simulink model "Soft_actuator_master_2021"  (R2020b)
settings: Solver=FixedStepAuto  StartTime=0.0  StopTime=inf  FixedStep=Ts  RelTol=1e-3  EnableMultiTasking=on
undefined symbols (not defined in the file or in its folder): Ts
libraries: arduinolib x6, simulink x2, pid_lib x1, dspfdesign x1
settings Model: SimulationMode=external  SILPILModeSetting=veronly  ExtModeTrigDuration=2  Creator=4D Lab  LastModifiedBy=Jakob Jansson
settings SolverCC: PositivePriorityOrder=on
settings OptimizationCC: EnhancedBackFolding=on  PassReuseOutputArgsAs=Individual arguments  ZeroExternalMemoryAtStartup=off  ZeroInternalMemoryAtStartup=off  MaxStackSize=64  OptimizeBlockOrder=speed  DifferentSizesBufferReuse=on  OptimizationCustomize=off  EfficientTunableParamExpr=on
settings DebuggingCC: ParameterTunabilityLossMsg=error
settings HardwareCC: ProdBitPerInt=16  ProdBitPerPointer=16  ProdBitPerSizeT=16  ProdBitPerPtrDiffT=16  ProdLargestAtomicFloat=None  ProdWordSize=8  ProdHWDeviceType=Atmel->AVR
settings RTWCC: Description=Embedded Coder  SystemTargetFile=ert.tlc  HardwareBoard=Arduino Mega 2560  TLCOptions="-aInlineSetEventsForThisBaseRateFcn=TLC_FALSE -aSuppressMultiTaskScheduler=TLC_FALSE   -aRateBasedStepFcn=1"  TemplateMakefile=ert_default_tmf  Toolchain=Arduino AVR  BuildConfiguration=Faster Runs
settings CodeAppCC: ForceParamTrailComments=on  IgnoreCustomStorageClasses=off  OperatorAnnotations=on  SimulinkDataObjDesc=on  SFDataObjDesc=on  InsertBlockDesc=on
settings ERTTargetCC: SupportContinuousTime=on  SupportVariableSizeSignals=on  ExtMode=on  ExtModeStaticAllocSize=2048  ExtModeMexArgs='127.0.0.1' 0 17725

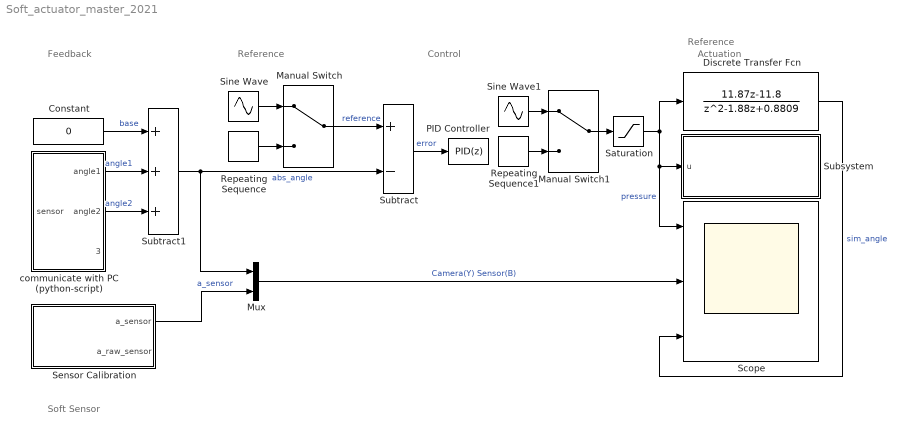
== system Soft_actuator_master_2021 ==
  note: Reference
  note: Feedback
  note: Soft Sensor
  note: Reference
  note: Actuation
  note: Control
  Constant : Constant  Value=0
  Discrete Transfer Fcn : DiscreteTransferFcn  Numerator=[11.87 -11.8]  Denominator=[1 -1.88 0.8809]
  Manual Switch : ManualSwitch
  Manual Switch1 : ManualSwitch
  Mux : Mux  Inputs=2
  PID Controller : pid_lib/PID Controller  Controller=PID  Form=Parallel  TimeDomain=Discrete-time  UseExternalTs=off  SampleTime=-1  IntegratorMethod=Forward Euler  FilterMethod=Forward Euler  ControllerParametersSource=internal  P=0.014114  I=0.11  D=-7.28e-05  UseFilter=on  N=25.7343  TunerSelectOption=Transfer Function Based (PID Tuner App)  InitialConditionSource=internal  InitialConditionForIntegrator=0  InitialConditionForFilter=0  DifferentiatorICPrevScaledInput=0  ExternalReset=none  TrackingMode=off  Kt=1  LimitOutput=off  SatLimitsSource=internal  UpperSaturationLimit=inf  LowerSaturationLimit=-inf  LinearizeAsGain=on  AntiWindupMode=none  Kb=1  POutMin=[]  POutMax=[]  IOutMin=[]  IOutMax=[]  DOutMin=[]  DOutMax=[]  NOutMin=[]  NOutMax=[]  SumOutMin=[]  SumOutMax=[]  SaturationOutMin=[]  SaturationOutMax=[]  PParamMin=[]  PParamMax=[]  IParamMin=[]  IParamMax=[]  DParamMin=[]  DParamMax=[]  NParamMin=[]  NParamMax=[]  KbParamMin=[]  KbParamMax=[]  KtParamMin=[]  KtParamMax=[]  KbOutMin=[]  KbOutMax=[]  KtOutMin=[]  KtOutMax=[]  IntegratorOutMin=[]  IntegratorOutMax=[]  FilterOutMin=[]  FilterOutMax=[]  SumI1OutMin=[]  SumI1OutMax=[]  SumI2OutMin=[]  SumI2OutMax=[]  SumI3OutMin=[]  SumI3OutMax=[]  SumI4OutMin=[]  SumI4OutMax=[]  SumDOutMin=[]  SumDOutMax=[]  DifferentiatorOutMin=[]  DifferentiatorOutMax=[]  FilterDiffOutCoefMin=[]  FilterDiffOutCoefMax=[]  ReciprocalOutMin=[]  ReciprocalOutMax=[]  SumDenOutMin=[]  SumDenOutMax=[]  SumNumOutMin=[]  SumNumOutMax=[]  DivideOutMin=[]  DivideOutMax=[]  UdiffTsProdOutMin=[]  UdiffTsProdOutMax=[]  NTsProdOutMin=[]  NTsProdOutMax=[]  UintegralTsProdOutMin=[]  UintegralTsProdOutMax=[]  UngainTsProdOutMin=[]  UngainTsProdOutMax=[]  IntegratorContinuousStateAttributes=''  IntegratorStateMustResolveToSignalObject=off  IntegratorRTWStateStorageClass=Auto  FilterContinuousStateAttributes=''  FilterStateMustResolveToSignalObject=off  FilterRTWStateStorageClass=Auto  ParallelPVariant=InternalParameters  IdealPVariant=Disabled  IVariant=InternalParameters  DVariant=InternalParameters  IntegratorVariant=Discrete  SatVariant=Disabled  AWVariant=Passthrough  PCopyVariant=Disabled  TRVariant=Disabled  FdbkBlocksVariant=Forward  IdealPFdbkVariant=Disabled  SatFdbkVariant=Disabled  DerivativeFilterVariant=ForwardEulerFilter  NVariant=InternalParameters  NCopyVariant=Disabled  FilterICVariant=InternalICsFilter  IntegratorICVariant=InternalICs  ExternalResetVariant=Disabled  TRSumVariant=Passthrough  SumFdbkVariant=Disabled  SumVariant=Sum_PID  TsampFilterVariant=InternalTs  TsampNgainVariant=Passthrough  TsampIntegralVariant=Passthrough  ExternalSaturationOutDataTypeStr=Inherit: Same as second input
  Repeating Sequence : simulink/Sources/Repeating Sequence  rep_seq_t=[0 4 6 10 12]  rep_seq_y=[0 0 180 180 0]
  Repeating Sequence1 : simulink/Sources/Repeating Sequence  rep_seq_t=[0 4 6 10 12]  rep_seq_y=[0 0 180 180 0]
  Saturation : Saturate  UpperLimit=6  LowerLimit=0
  Scope : Scope  NumInputPorts=3
  Sensor Calibration : Subsystem
  Sine Wave : Sin  Amplitude=45  Bias=135  SampleTime=Ts
  Sine Wave1 : Sin  Bias=1  Frequency=2  SampleTime=Ts
  Subsystem : Subsystem
  Subtract : Sum  Inputs=+-
  Subtract1 : Sum  Inputs=+++
  communicate with PC (python-script) : Subsystem
  wires:
  Subtract1/1 -> Subtract/2, Mux/1  "abs_angle"
  Subtract/1 -> PID Controller/1  "error"
  Sine Wave/1 -> Manual Switch/1
  Repeating Sequence/1 -> Manual Switch/2
  Manual Switch/1 -> Subtract/1  "reference"
  communicate with PC (python-script)/2(angle2) -> Subtract1/3  "angle2"
  communicate with PC (python-script)/1(angle1) -> Subtract1/2  "angle1"
  Constant/1 -> Subtract1/1  "base"
  Discrete Transfer Fcn/1 -> Scope/3  "sim_angle"
  Manual Switch1/1 -> Saturation/1
  Saturation/1 -> Discrete Transfer Fcn/1, Scope/1, Subsystem/1(u)  "pressure"
  Sensor Calibration/1(a_sensor) -> Mux/2  "a_sensor"
  Mux/1 -> Scope/2  "Camera(Y) Sensor(B)"
  Repeating Sequence1/1 -> Manual Switch1/2
  Sine Wave1/1 -> Manual Switch1/1

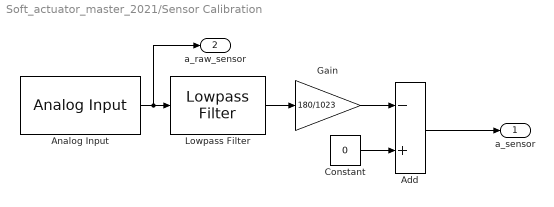
== system Soft_actuator_master_2021/Sensor Calibration ==
  Add : Sum  Inputs=-+
  Analog Input : arduinolib/Analog Input  pinNumber=4  ReadResultsOnly=off  ConversionTriggerSource=Software  ExternalTriggerType=uint32( 0 )  OutputDataType=uint16  EnableConversionCompleteNotify=off  EnableOuputStatus=off  SampleTime=Ts  blockPlatform=arduino
  Constant : Constant  Value=0
  Gain : Gain  Gain=180/1023
  Lowpass Filter : dspfdesign/Lowpass Filter  FilterType=FIR  DesignForMinimumOrder=on  FilterOrder=50  PassbandFrequency=8e3  StopbandFrequency=12e3  PassbandRipple=0.1  StopbandAttenuation=80  InheritSampleRate=off  SampleRate=44100  SimulateUsing=Interpreted execution  roundingMode=Floor  coeffsDataTypeStr=fixdt(1,16)
  a_sensor : Outport
  a_raw_sensor : Outport  Port=2
  wires:
  Gain/1 -> Add/1
  Constant/1 -> Add/2
  Analog Input/1 -> a_raw_sensor/1, Lowpass Filter/1
  Lowpass Filter/1 -> Gain/1
  Add/1 -> a_sensor/1

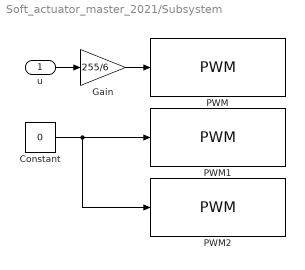
== system Soft_actuator_master_2021/Subsystem ==
  u : Inport
  Constant : Constant  Value=0
  Gain : Gain  Gain=255/6
  PWM : arduinolib/PWM  pinNumber=3  frequencyType=Default  desiredFrequency=490.2  achievableFrequency=490.2
  PWM1 : arduinolib/PWM  pinNumber=5  frequencyType=Default  desiredFrequency=490.2  achievableFrequency=490.2
  PWM2 : arduinolib/PWM  pinNumber=6  frequencyType=Default  desiredFrequency=490.2  achievableFrequency=490.2
  wires:
  Gain/1 -> PWM/1
  u/1 -> Gain/1
  Constant/1 -> PWM1/1, PWM2/1

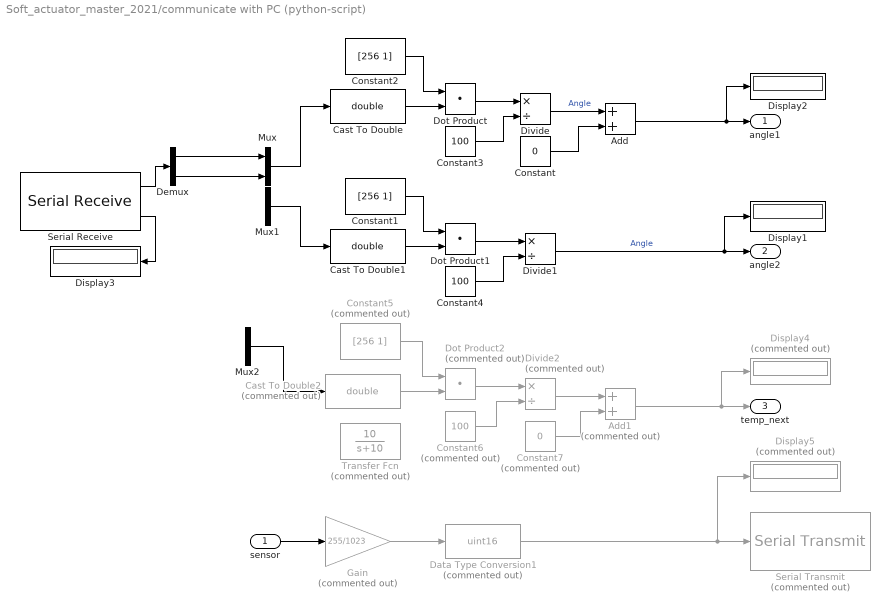
== system Soft_actuator_master_2021/communicate with PC (python-script) ==
  sensor : Inport
  Add : Sum
  Add1 : Sum  Commented=on
  Cast To Double : DataTypeConversion  OutDataTypeStr=double
  Cast To Double1 : DataTypeConversion  OutDataTypeStr=double
  Cast To Double2 : DataTypeConversion  Commented=on  OutDataTypeStr=double
  Constant : Constant  Value=0
  Constant1 : Constant  Value=[256 1]
  Constant2 : Constant  Value=[256 1]
  Constant3 : Constant  Value=100
  Constant4 : Constant  Value=100
  Constant5 : Constant  Commented=on  Value=[256 1]  OutDataTypeStr=double
  Constant6 : Constant  Commented=on  Value=100
  Constant7 : Constant  Commented=on  Value=0
  Data Type Conversion1 : DataTypeConversion  Commented=on  OutDataTypeStr=uint16
  Demux : Demux  Outputs=2
  Display1 : Display
  Display2 : Display
  Display3 : Display
  Display4 : Display  Commented=on
  Display5 : Display  Commented=on
  Divide : Product  Inputs=*/
  Divide1 : Product  Inputs=*/
  Divide2 : Product  Commented=on  Inputs=*/  OutDataTypeStr=double
  Dot Product : DotProduct  InputSameDT=on  OutDataTypeStr=Inherit: Inherit via internal rule
  Dot Product1 : DotProduct  InputSameDT=on  OutDataTypeStr=Inherit: Inherit via internal rule
  Dot Product2 : DotProduct  Commented=on  OutDataTypeStr=double  InputSameDT=on
  Gain : Gain  Commented=on  Gain=255/1023  ParamDataTypeStr=uint16
  Mux : Mux  Inputs=2
  Mux1 : Mux  Inputs=2
  Mux2 : Mux  Inputs=2
  Serial Receive : arduinolib/Serial Receive  isARMArch=off  portNumber=1  DataType=uint8  Datalength=2  SampleTime=Ts  showOutStatus=on  blockPlatform=arduino
      settings: SourceProductBaseCode=ARDUINO
  Serial Transmit : arduinolib/Serial Transmit  Commented=on  portNumber=1  sendmode=println  sendformat=Decimal  floatprecision=2  blockPlatform=arduino
  Transfer Fcn : TransferFcn  Commented=on  Numerator=[10]  Denominator=[1 10]
  angle1 : Outport  VectorParamsAs1DForOutWhenUnconnected=off
  angle2 : Outport  Port=2  VectorParamsAs1DForOutWhenUnconnected=off
  temp_next : Outport  Port=3  VectorParamsAs1DForOutWhenUnconnected=off
  wires:
  Constant3/1 -> Divide/2
  Cast To Double/1 -> Dot Product/2
  Constant2/1 -> Dot Product/1
  Dot Product/1 -> Divide/1
  Serial Receive/1 -> Demux/1
  Demux/1 -> Mux/1
  Demux/2 -> Mux/2
  Dot Product1/1 -> Divide1/1
  Constant4/1 -> Divide1/2
  Cast To Double1/1 -> Dot Product1/2
  Constant1/1 -> Dot Product1/1
  Mux/1 -> Cast To Double/1
  Mux1/1 -> Cast To Double1/1
  Divide1/1 -> Display1/1, angle2/1  "Angle"
  Serial Receive/2 -> Display3/1
  Cast To Double2/1 -> Dot Product2/2
  Constant5/1 -> Dot Product2/1
  Constant6/1 -> Divide2/2
  Mux2/1 -> Cast To Double2/1
  Dot Product2/1 -> Divide2/1
  Data Type Conversion1/1 -> Display5/1, Serial Transmit/1
  Gain/1 -> Data Type Conversion1/1
  Constant/1 -> Add/2
  Divide/1 -> Add/1  "Angle"
  Add/1 -> Display2/1, angle1/1
  Divide2/1 -> Add1/1
  Constant7/1 -> Add1/2
  Add1/1 -> Display4/1, temp_next/1
  sensor/1 -> Gain/1
